simulink model "TST_ACSwt_VD"  (R2016b)
settings: Solver=FixedStepDiscrete  StartTime=0.0  StopTime=simTime  FixedStep=sampleTime  RelTol=1e-3
values from neighbouring files (symbols this model uses):
  testCase = 1    [initTST_ACSwt_VD_001.m]    (also in initTST_ACSwt_VD_002.m = 2; initTST_ACSwt_VD_003.m = 3; initTST_ACSwt_VD_004.m = 4)
libraries: simulink x9, UnitTest_Lib x4
settings Model: Creator=zhengjinyan  LastModifiedBy=zhengjinyan
settings DebuggingCC: SignalRangeChecking=error

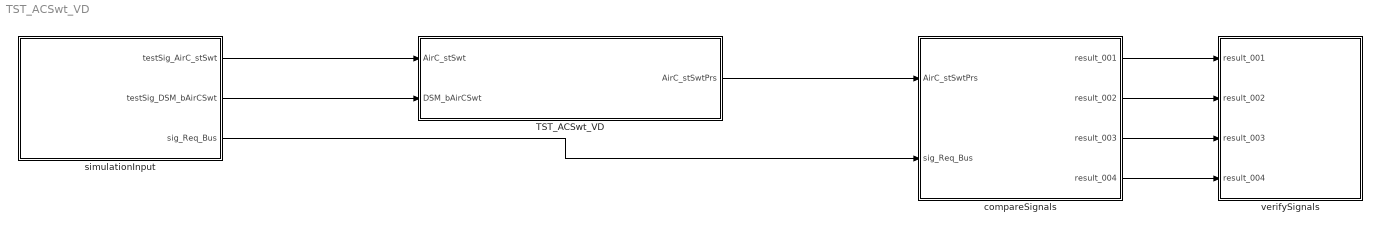
== system TST_ACSwt_VD ==
  TST_ACSwt_VD : Subsystem
  compareSignals : Subsystem
  simulationInput : Subsystem
  verifySignals : Subsystem
  wires:
  simulationInput/1(testSig_AirC_stSwt) -> TST_ACSwt_VD/1(AirC_stSwt)
  simulationInput/2(testSig_DSM_bAirCSwt) -> TST_ACSwt_VD/2(DSM_bAirCSwt)
  TST_ACSwt_VD/1(AirC_stSwtPrs) -> compareSignals/1(AirC_stSwtPrs)
  simulationInput/3(sig_Req_Bus) -> compareSignals/2(sig_Req_Bus)
  compareSignals/1(result_001) -> verifySignals/1(result_001)
  compareSignals/2(result_002) -> verifySignals/2(result_002)
  compareSignals/3(result_003) -> verifySignals/3(result_003)
  compareSignals/4(result_004) -> verifySignals/4(result_004)

== system TST_ACSwt_VD/TST_ACSwt_VD ==
  AirC_stSwt : Inport
  DSM_bAirCSwt : Inport  Port=2
  ACSwt_VD : ModelReference  ModelNameDialog=ACSwt_VD  SimulationMode=Normal  ModelReferenceVersion=1.10  TriggerPortName=function  TriggerPortTriggerType=function-call  TriggerPortStatesWhenEnabling=held
  Function_Call : simulink/Ports & Subsystems/Function-Call Generator  sample_time=sampleTime  numberOfIterations=1
  AirC_stSwtPrs : Outport
  wires:
  Function_Call/1 -> ACSwt_VD/Trigger
  AirC_stSwt/1 -> ACSwt_VD/1
  DSM_bAirCSwt/1 -> ACSwt_VD/2
  ACSwt_VD/1 -> AirC_stSwtPrs/1

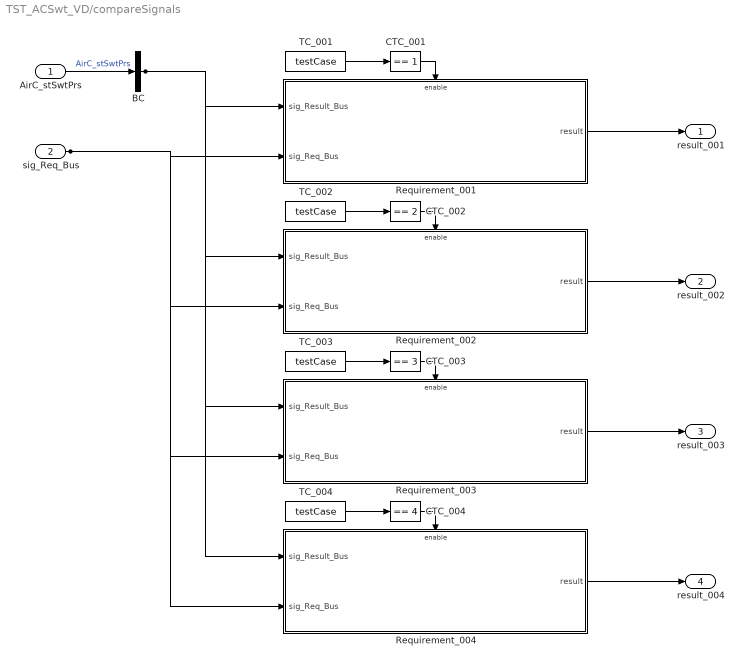
== system TST_ACSwt_VD/compareSignals ==
  AirC_stSwtPrs : Inport
  sig_Req_Bus : Inport  Port=2
  BC : BusCreator  Inputs=1
  CTC_001 : simulink/Logic and Bit Operations/Compare To Constant  relop===  const=1  OutDataTypeStr=boolean
  CTC_002 : simulink/Logic and Bit Operations/Compare To Constant  relop===  const=2  OutDataTypeStr=boolean
  CTC_003 : simulink/Logic and Bit Operations/Compare To Constant  relop===  const=3  OutDataTypeStr=boolean
  CTC_004 : simulink/Logic and Bit Operations/Compare To Constant  relop===  const=4  OutDataTypeStr=boolean
  Requirement_001 : Subsystem
  Requirement_002 : Subsystem
  Requirement_003 : Subsystem
  Requirement_004 : Subsystem
  TC_001 : Constant  Value=testCase
  TC_002 : Constant  Value=testCase
  TC_003 : Constant  Value=testCase
  TC_004 : Constant  Value=testCase
  result_001 : Outport
  result_002 : Outport  Port=2
  result_003 : Outport  Port=3
  result_004 : Outport  Port=4
  wires:
  AirC_stSwtPrs/1 -> BC/1  "AirC_stSwtPrs"
  TC_001/1 -> CTC_001/1
  CTC_001/1 -> Requirement_001/Enable
  sig_Req_Bus/1 -> Requirement_001/2(sig_Req_Bus), Requirement_002/2(sig_Req_Bus), Requirement_003/2(sig_Req_Bus), Requirement_004/2(sig_Req_Bus)
  BC/1 -> Requirement_001/1(sig_Result_Bus), Requirement_002/1(sig_Result_Bus), Requirement_003/1(sig_Result_Bus), Requirement_004/1(sig_Result_Bus)
  Requirement_001/1(result) -> result_001/1
  TC_002/1 -> CTC_002/1
  CTC_002/1 -> Requirement_002/Enable
  Requirement_002/1(result) -> result_002/1
  TC_003/1 -> CTC_003/1
  CTC_003/1 -> Requirement_003/Enable
  Requirement_003/1(result) -> result_003/1
  TC_004/1 -> CTC_004/1
  CTC_004/1 -> Requirement_004/Enable
  Requirement_004/1(result) -> result_004/1

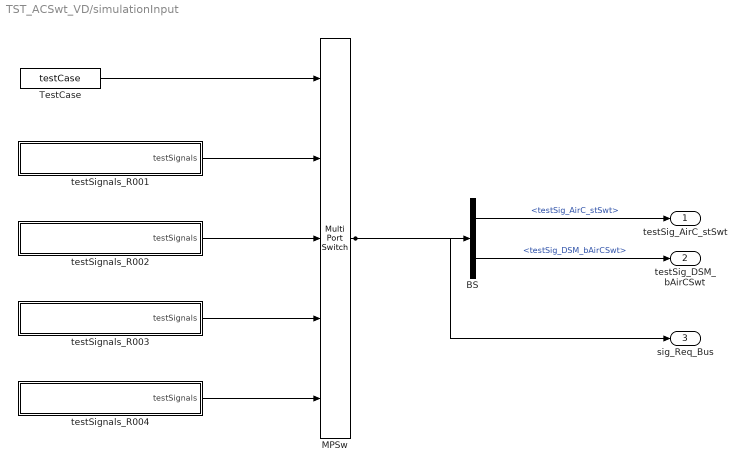
== system TST_ACSwt_VD/simulationInput ==
  BS : BusSelector  OutputSignals=testSig_AirC_stSwt,testSig_DSM_bAirCSwt
  MPSw : MultiPortSwitch  Inputs=4  SaturateOnIntegerOverflow=on  InputSameDT=on
  TestCase : Constant  Value=testCase
  testSignals_R001 : Subsystem
  testSignals_R002 : Subsystem
  testSignals_R003 : Subsystem
  testSignals_R004 : Subsystem
  testSig_AirC_stSwt : Outport
  testSig_DSM_bAirCSwt : Outport  Port=2
  sig_Req_Bus : Outport  Port=3
  wires:
  BS/1 -> testSig_AirC_stSwt/1  "<testSig_AirC_stSwt>"
  BS/2 -> testSig_DSM_bAirCSwt/1  "<testSig_DSM_bAirCSwt>"
  MPSw/1 -> BS/1, sig_Req_Bus/1
  TestCase/1 -> MPSw/1
  testSignals_R001/1(testSignals) -> MPSw/2
  testSignals_R002/1(testSignals) -> MPSw/3
  testSignals_R003/1(testSignals) -> MPSw/4
  testSignals_R004/1(testSignals) -> MPSw/5

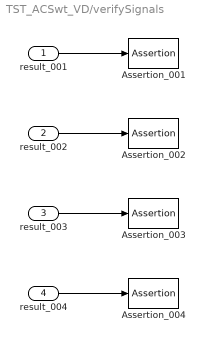
== system TST_ACSwt_VD/verifySignals ==
  result_001 : Inport
  result_002 : Inport  Port=2
  result_003 : Inport  Port=3
  result_004 : Inport  Port=4
  Assertion_001 : Assertion  Enabled=off
  Assertion_002 : Assertion  Enabled=off
  Assertion_003 : Assertion  Enabled=off
  Assertion_004 : Assertion  Enabled=off
  wires:
  result_001/1 -> Assertion_001/1
  result_002/1 -> Assertion_002/1
  result_003/1 -> Assertion_003/1
  result_004/1 -> Assertion_004/1

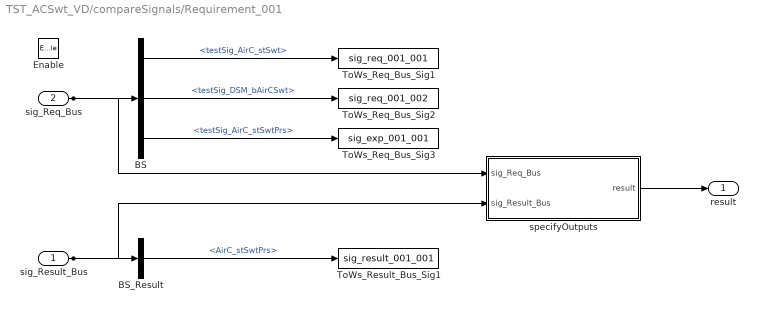
== system TST_ACSwt_VD/compareSignals/Requirement_001 ==
  sig_Result_Bus : Inport
  sig_Req_Bus : Inport  Port=2
  Enable : EnablePort
  BS : BusSelector  OutputSignals=testSig_AirC_stSwt,testSig_DSM_bAirCSwt,testSig_AirC_stSwtPrs
  BS_Result : BusSelector  OutputSignals=AirC_stSwtPrs
  ToWs_Req_Bus_Sig1 : ToWorkspace  VariableName=sig_req_001_001  SaveFormat=Structure With Time
  ToWs_Req_Bus_Sig2 : ToWorkspace  VariableName=sig_req_001_002  SaveFormat=Structure With Time
  ToWs_Req_Bus_Sig3 : ToWorkspace  VariableName=sig_exp_001_001  SaveFormat=Structure With Time
  ToWs_Result_Bus_Sig1 : ToWorkspace  VariableName=sig_result_001_001  SaveFormat=Structure With Time
  specifyOutputs : Subsystem
  result : Outport
  wires:
  sig_Req_Bus/1 -> BS/1, specifyOutputs/1(sig_Req_Bus)
  BS/1 -> ToWs_Req_Bus_Sig1/1  "<testSig_AirC_stSwt>"
  BS/2 -> ToWs_Req_Bus_Sig2/1  "<testSig_DSM_bAirCSwt>"
  BS/3 -> ToWs_Req_Bus_Sig3/1  "<testSig_AirC_stSwtPrs>"
  sig_Result_Bus/1 -> BS_Result/1, specifyOutputs/2(sig_Result_Bus)
  BS_Result/1 -> ToWs_Result_Bus_Sig1/1  "<AirC_stSwtPrs>"
  specifyOutputs/1(result) -> result/1

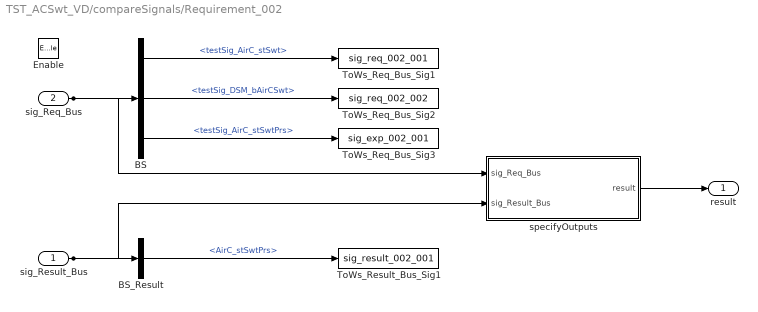
== system TST_ACSwt_VD/compareSignals/Requirement_002 ==
  sig_Result_Bus : Inport
  sig_Req_Bus : Inport  Port=2
  Enable : EnablePort
  BS : BusSelector  OutputSignals=testSig_AirC_stSwt,testSig_DSM_bAirCSwt,testSig_AirC_stSwtPrs
  BS_Result : BusSelector  OutputSignals=AirC_stSwtPrs
  ToWs_Req_Bus_Sig1 : ToWorkspace  VariableName=sig_req_002_001  SaveFormat=Structure With Time
  ToWs_Req_Bus_Sig2 : ToWorkspace  VariableName=sig_req_002_002  SaveFormat=Structure With Time
  ToWs_Req_Bus_Sig3 : ToWorkspace  VariableName=sig_exp_002_001  SaveFormat=Structure With Time
  ToWs_Result_Bus_Sig1 : ToWorkspace  VariableName=sig_result_002_001  SaveFormat=Structure With Time
  specifyOutputs : Subsystem
  result : Outport
  wires:
  sig_Req_Bus/1 -> BS/1, specifyOutputs/1(sig_Req_Bus)
  BS/1 -> ToWs_Req_Bus_Sig1/1  "<testSig_AirC_stSwt>"
  BS/2 -> ToWs_Req_Bus_Sig2/1  "<testSig_DSM_bAirCSwt>"
  BS/3 -> ToWs_Req_Bus_Sig3/1  "<testSig_AirC_stSwtPrs>"
  sig_Result_Bus/1 -> BS_Result/1, specifyOutputs/2(sig_Result_Bus)
  BS_Result/1 -> ToWs_Result_Bus_Sig1/1  "<AirC_stSwtPrs>"
  specifyOutputs/1(result) -> result/1

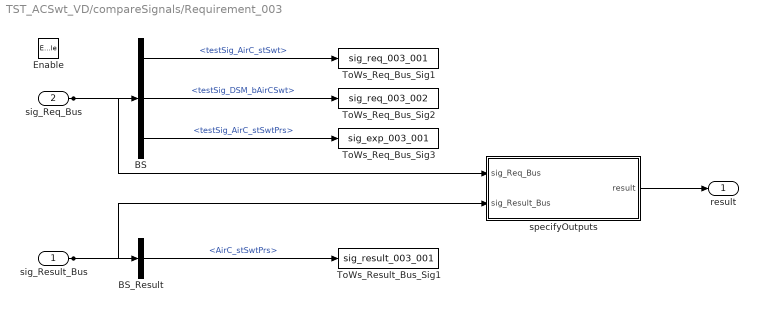
== system TST_ACSwt_VD/compareSignals/Requirement_003 ==
  sig_Result_Bus : Inport
  sig_Req_Bus : Inport  Port=2
  Enable : EnablePort
  BS : BusSelector  OutputSignals=testSig_AirC_stSwt,testSig_DSM_bAirCSwt,testSig_AirC_stSwtPrs
  BS_Result : BusSelector  OutputSignals=AirC_stSwtPrs
  ToWs_Req_Bus_Sig1 : ToWorkspace  VariableName=sig_req_003_001  SaveFormat=Structure With Time
  ToWs_Req_Bus_Sig2 : ToWorkspace  VariableName=sig_req_003_002  SaveFormat=Structure With Time
  ToWs_Req_Bus_Sig3 : ToWorkspace  VariableName=sig_exp_003_001  SaveFormat=Structure With Time
  ToWs_Result_Bus_Sig1 : ToWorkspace  VariableName=sig_result_003_001  SaveFormat=Structure With Time
  specifyOutputs : Subsystem
  result : Outport
  wires:
  sig_Req_Bus/1 -> BS/1, specifyOutputs/1(sig_Req_Bus)
  BS/1 -> ToWs_Req_Bus_Sig1/1  "<testSig_AirC_stSwt>"
  BS/2 -> ToWs_Req_Bus_Sig2/1  "<testSig_DSM_bAirCSwt>"
  BS/3 -> ToWs_Req_Bus_Sig3/1  "<testSig_AirC_stSwtPrs>"
  sig_Result_Bus/1 -> BS_Result/1, specifyOutputs/2(sig_Result_Bus)
  BS_Result/1 -> ToWs_Result_Bus_Sig1/1  "<AirC_stSwtPrs>"
  specifyOutputs/1(result) -> result/1

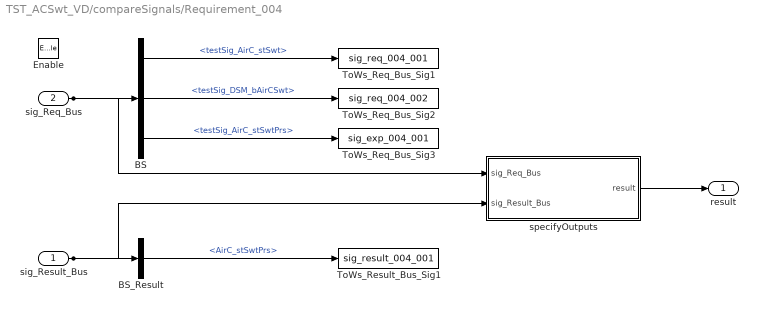
== system TST_ACSwt_VD/compareSignals/Requirement_004 ==
  sig_Result_Bus : Inport
  sig_Req_Bus : Inport  Port=2
  Enable : EnablePort
  BS : BusSelector  OutputSignals=testSig_AirC_stSwt,testSig_DSM_bAirCSwt,testSig_AirC_stSwtPrs
  BS_Result : BusSelector  OutputSignals=AirC_stSwtPrs
  ToWs_Req_Bus_Sig1 : ToWorkspace  VariableName=sig_req_004_001  SaveFormat=Structure With Time
  ToWs_Req_Bus_Sig2 : ToWorkspace  VariableName=sig_req_004_002  SaveFormat=Structure With Time
  ToWs_Req_Bus_Sig3 : ToWorkspace  VariableName=sig_exp_004_001  SaveFormat=Structure With Time
  ToWs_Result_Bus_Sig1 : ToWorkspace  VariableName=sig_result_004_001  SaveFormat=Structure With Time
  specifyOutputs : Subsystem
  result : Outport
  wires:
  sig_Req_Bus/1 -> BS/1, specifyOutputs/1(sig_Req_Bus)
  BS/1 -> ToWs_Req_Bus_Sig1/1  "<testSig_AirC_stSwt>"
  BS/2 -> ToWs_Req_Bus_Sig2/1  "<testSig_DSM_bAirCSwt>"
  BS/3 -> ToWs_Req_Bus_Sig3/1  "<testSig_AirC_stSwtPrs>"
  sig_Result_Bus/1 -> BS_Result/1, specifyOutputs/2(sig_Result_Bus)
  BS_Result/1 -> ToWs_Result_Bus_Sig1/1  "<AirC_stSwtPrs>"
  specifyOutputs/1(result) -> result/1

== system TST_ACSwt_VD/simulationInput/testSignals_R001 ==
  BC : BusCreator  Inputs=3
  spec_AirC_stSwt : FromWorkspace  VariableName=testSig_AirC_stSwt  Interpolate=off  OutputAfterFinalValue=Holding final value
  spec_AirC_stSwtPrs : FromWorkspace  VariableName=testSig_AirC_stSwtPrs  Interpolate=off  OutputAfterFinalValue=Holding final value
  spec_DSM_bAirCSwt : FromWorkspace  VariableName=testSig_DSM_bAirCSwt  Interpolate=off  OutputAfterFinalValue=Holding final value
  testSignals : Outport
  wires:
  BC/1 -> testSignals/1
  spec_AirC_stSwt/1 -> BC/1  "testSig_AirC_stSwt"
  spec_DSM_bAirCSwt/1 -> BC/2  "testSig_DSM_bAirCSwt"
  spec_AirC_stSwtPrs/1 -> BC/3  "testSig_AirC_stSwtPrs"

== system TST_ACSwt_VD/simulationInput/testSignals_R002 ==
  BC : BusCreator  Inputs=3
  spec_AirC_stSwt : FromWorkspace  VariableName=testSig_AirC_stSwt  Interpolate=off  OutputAfterFinalValue=Holding final value
  spec_AirC_stSwtPrs : FromWorkspace  VariableName=testSig_AirC_stSwtPrs  Interpolate=off  OutputAfterFinalValue=Holding final value
  spec_DSM_bAirCSwt : FromWorkspace  VariableName=testSig_DSM_bAirCSwt  Interpolate=off  OutputAfterFinalValue=Holding final value
  testSignals : Outport
  wires:
  BC/1 -> testSignals/1
  spec_AirC_stSwt/1 -> BC/1  "testSig_AirC_stSwt"
  spec_DSM_bAirCSwt/1 -> BC/2  "testSig_DSM_bAirCSwt"
  spec_AirC_stSwtPrs/1 -> BC/3  "testSig_AirC_stSwtPrs"

== system TST_ACSwt_VD/simulationInput/testSignals_R003 ==
  BC : BusCreator  Inputs=3
  spec_AirC_stSwt : FromWorkspace  VariableName=testSig_AirC_stSwt  Interpolate=off  OutputAfterFinalValue=Holding final value
  spec_AirC_stSwtPrs : FromWorkspace  VariableName=testSig_AirC_stSwtPrs  Interpolate=off  OutputAfterFinalValue=Holding final value
  spec_DSM_bAirCSwt : FromWorkspace  VariableName=testSig_DSM_bAirCSwt  Interpolate=off  OutputAfterFinalValue=Holding final value
  testSignals : Outport
  wires:
  BC/1 -> testSignals/1
  spec_AirC_stSwt/1 -> BC/1  "testSig_AirC_stSwt"
  spec_DSM_bAirCSwt/1 -> BC/2  "testSig_DSM_bAirCSwt"
  spec_AirC_stSwtPrs/1 -> BC/3  "testSig_AirC_stSwtPrs"

== system TST_ACSwt_VD/simulationInput/testSignals_R004 ==
  BC : BusCreator  Inputs=3
  spec_AirC_stSwt : FromWorkspace  VariableName=testSig_AirC_stSwt  Interpolate=off  OutputAfterFinalValue=Holding final value
  spec_AirC_stSwtPrs : FromWorkspace  VariableName=testSig_AirC_stSwtPrs  Interpolate=off  OutputAfterFinalValue=Holding final value
  spec_DSM_bAirCSwt : FromWorkspace  VariableName=testSig_DSM_bAirCSwt  Interpolate=off  OutputAfterFinalValue=Holding final value
  testSignals : Outport
  wires:
  BC/1 -> testSignals/1
  spec_AirC_stSwt/1 -> BC/1  "testSig_AirC_stSwt"
  spec_DSM_bAirCSwt/1 -> BC/2  "testSig_DSM_bAirCSwt"
  spec_AirC_stSwtPrs/1 -> BC/3  "testSig_AirC_stSwtPrs"

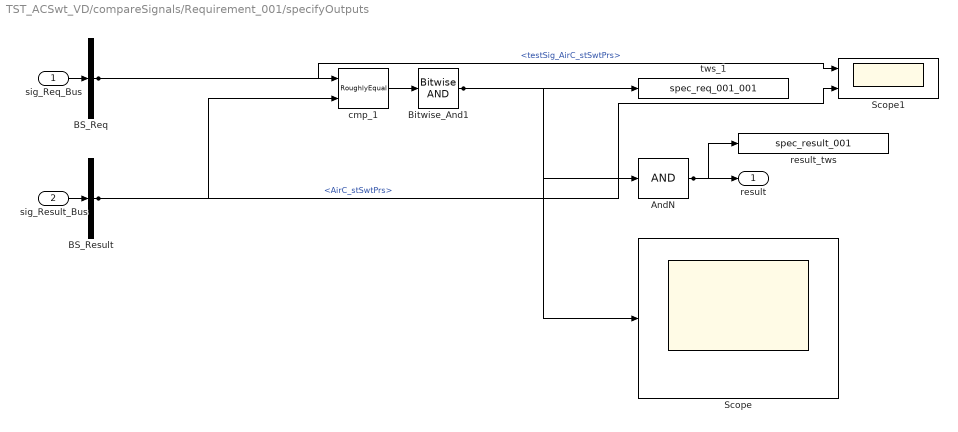
== system TST_ACSwt_VD/compareSignals/Requirement_001/specifyOutputs ==
  sig_Req_Bus : Inport
  sig_Result_Bus : Inport  Port=2
  AndN : Logic  Inputs=1
  BS_Req : BusSelector  OutputSignals=testSig_AirC_stSwtPrs
  BS_Result : BusSelector  OutputSignals=AirC_stSwtPrs
  Bitwise_And1 : simulink/Logic and Bit Operations/Bitwise Operator  logicop=AND  UseBitMask=off  BitMask=bin2dec('11011001')  BitMaskRealWorld=Stored Integer
  Scope : Scope
  Scope1 : Scope  NumInputPorts=2
  cmp_1 : UnitTest_Lib/RoughlyEqual  slope=0.1
  result_tws : ToWorkspace  VariableName=spec_result_001
  tws_1 : ToWorkspace  VariableName=spec_req_001_001
  result : Outport
  wires:
  sig_Req_Bus/1 -> BS_Req/1
  sig_Result_Bus/1 -> BS_Result/1
  AndN/1 -> result/1, result_tws/1
  BS_Req/1 -> cmp_1/1, Scope1/1  "<testSig_AirC_stSwtPrs>"
  BS_Result/1 -> cmp_1/2, Scope1/2  "<AirC_stSwtPrs>"
  cmp_1/1 -> Bitwise_And1/1
  Bitwise_And1/1 -> tws_1/1, AndN/1, Scope/1

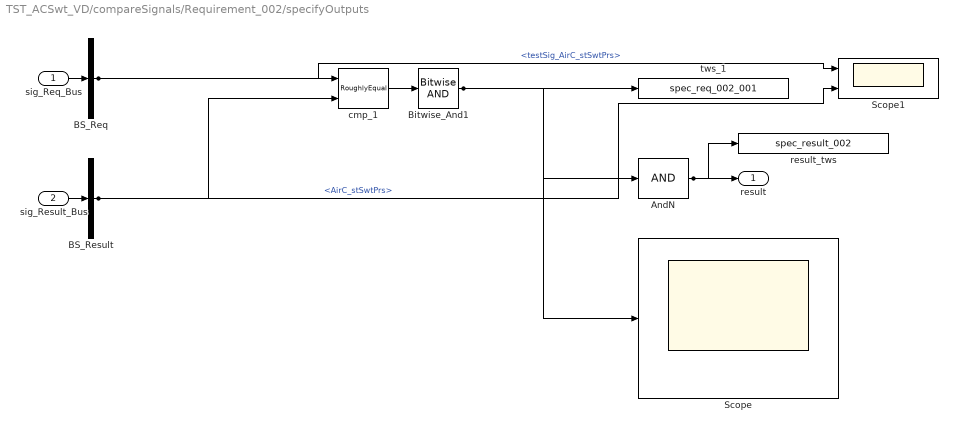
== system TST_ACSwt_VD/compareSignals/Requirement_002/specifyOutputs ==
  sig_Req_Bus : Inport
  sig_Result_Bus : Inport  Port=2
  AndN : Logic  Inputs=1
  BS_Req : BusSelector  OutputSignals=testSig_AirC_stSwtPrs
  BS_Result : BusSelector  OutputSignals=AirC_stSwtPrs
  Bitwise_And1 : simulink/Logic and Bit Operations/Bitwise Operator  logicop=AND  UseBitMask=off  BitMask=bin2dec('11011001')  BitMaskRealWorld=Stored Integer
  Scope : Scope
  Scope1 : Scope  NumInputPorts=2
  cmp_1 : UnitTest_Lib/RoughlyEqual  slope=0.1
  result_tws : ToWorkspace  VariableName=spec_result_002
  tws_1 : ToWorkspace  VariableName=spec_req_002_001
  result : Outport
  wires:
  sig_Req_Bus/1 -> BS_Req/1
  sig_Result_Bus/1 -> BS_Result/1
  AndN/1 -> result/1, result_tws/1
  BS_Req/1 -> cmp_1/1, Scope1/1  "<testSig_AirC_stSwtPrs>"
  BS_Result/1 -> cmp_1/2, Scope1/2  "<AirC_stSwtPrs>"
  cmp_1/1 -> Bitwise_And1/1
  Bitwise_And1/1 -> tws_1/1, AndN/1, Scope/1

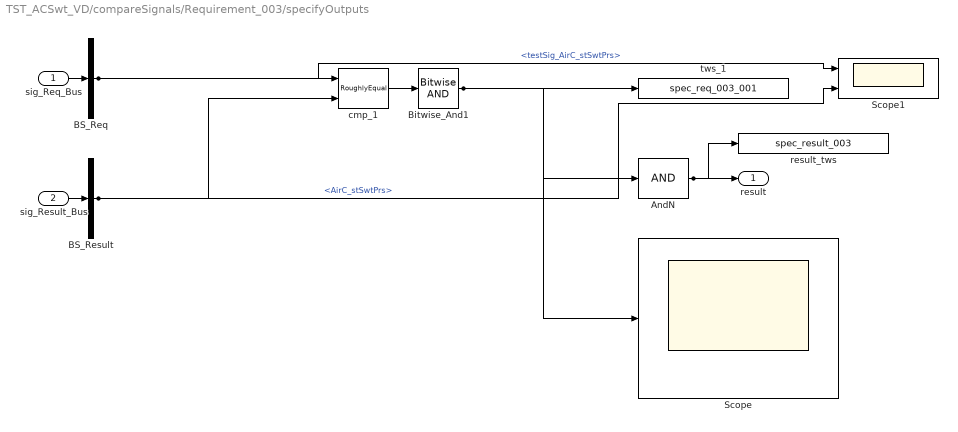
== system TST_ACSwt_VD/compareSignals/Requirement_003/specifyOutputs ==
  sig_Req_Bus : Inport
  sig_Result_Bus : Inport  Port=2
  AndN : Logic  Inputs=1
  BS_Req : BusSelector  OutputSignals=testSig_AirC_stSwtPrs
  BS_Result : BusSelector  OutputSignals=AirC_stSwtPrs
  Bitwise_And1 : simulink/Logic and Bit Operations/Bitwise Operator  logicop=AND  UseBitMask=off  BitMask=bin2dec('11011001')  BitMaskRealWorld=Stored Integer
  Scope : Scope
  Scope1 : Scope  NumInputPorts=2
  cmp_1 : UnitTest_Lib/RoughlyEqual  slope=0.1
  result_tws : ToWorkspace  VariableName=spec_result_003
  tws_1 : ToWorkspace  VariableName=spec_req_003_001
  result : Outport
  wires:
  sig_Req_Bus/1 -> BS_Req/1
  sig_Result_Bus/1 -> BS_Result/1
  AndN/1 -> result/1, result_tws/1
  BS_Req/1 -> cmp_1/1, Scope1/1  "<testSig_AirC_stSwtPrs>"
  BS_Result/1 -> cmp_1/2, Scope1/2  "<AirC_stSwtPrs>"
  cmp_1/1 -> Bitwise_And1/1
  Bitwise_And1/1 -> tws_1/1, AndN/1, Scope/1

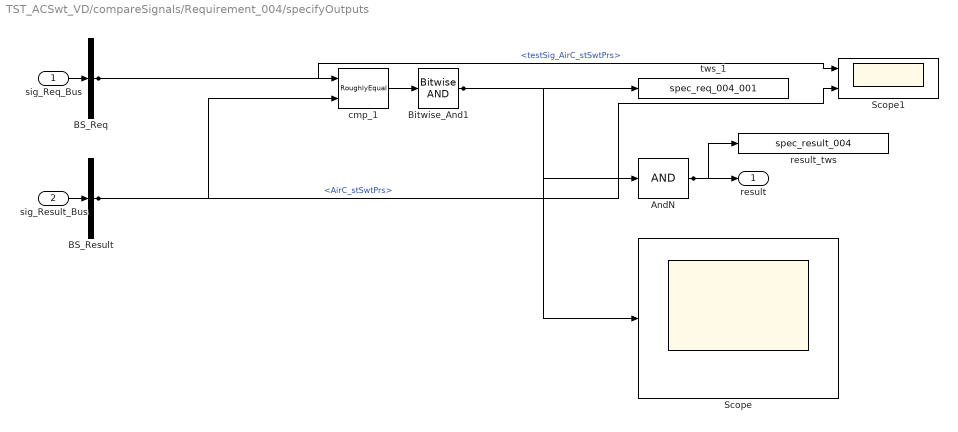
== system TST_ACSwt_VD/compareSignals/Requirement_004/specifyOutputs ==
  sig_Req_Bus : Inport
  sig_Result_Bus : Inport  Port=2
  AndN : Logic  Inputs=1
  BS_Req : BusSelector  OutputSignals=testSig_AirC_stSwtPrs
  BS_Result : BusSelector  OutputSignals=AirC_stSwtPrs
  Bitwise_And1 : simulink/Logic and Bit Operations/Bitwise Operator  logicop=AND  UseBitMask=off  BitMask=bin2dec('11011001')  BitMaskRealWorld=Stored Integer
  Scope : Scope
  Scope1 : Scope  NumInputPorts=2
  cmp_1 : UnitTest_Lib/RoughlyEqual  slope=0.1
  result_tws : ToWorkspace  VariableName=spec_result_004
  tws_1 : ToWorkspace  VariableName=spec_req_004_001
  result : Outport
  wires:
  sig_Req_Bus/1 -> BS_Req/1
  sig_Result_Bus/1 -> BS_Result/1
  AndN/1 -> result/1, result_tws/1
  BS_Req/1 -> cmp_1/1, Scope1/1  "<testSig_AirC_stSwtPrs>"
  BS_Result/1 -> cmp_1/2, Scope1/2  "<AirC_stSwtPrs>"
  cmp_1/1 -> Bitwise_And1/1
  Bitwise_And1/1 -> tws_1/1, AndN/1, Scope/1
